simulink model "second_order_DDPG_change_obs"  (R2024a)
settings: Solver=FixedStepAuto  StartTime=0.0  StopTime=500  FixedStep=0.001  RelTol=1e-3
libraries: rllib x1, simulink x1
settings Model: Creator=Steven  LastModifiedBy=Steven
settings DebuggingCC: UnconnectedInputMsg=warning  UnconnectedOutputMsg=warning  UnconnectedLineMsg=warning
settings ModelReferenceCC: EnableRefExpFcnMdlSchedulingChecks=on
settings RTWCC: GPUComputeCapability=3.5  DLArmComputeVersion=19.05

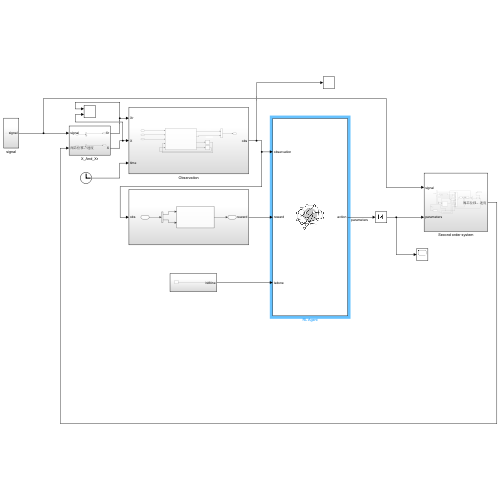
[thumbnail: Simulink's stored preview of the top-level diagram]
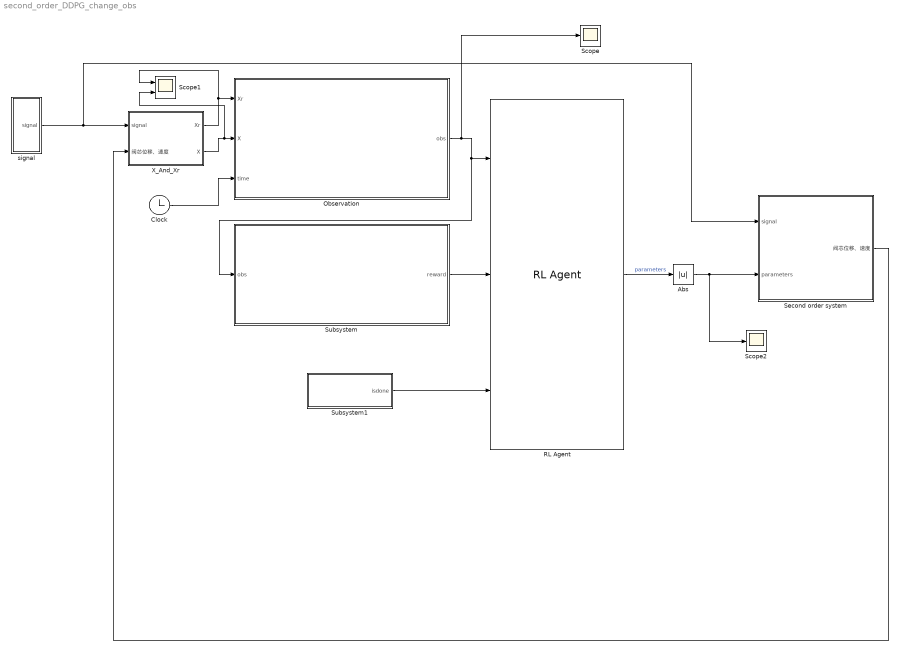
== system second_order_DDPG_change_obs ==
  Abs : Abs  SaturateOnIntegerOverflow=off
  Clock : Clock
  Observation : Subsystem
  RL Agent : rllib/RL Agent  Agent=agent_second_order  ExternalActionAsInput=off  ProvideLastAction=off  ProvideCumRwd=off  TreatAsDirectFeedthrough=on  UseStrictObservationDataTypes=off
  Scope : Scope
  Scope1 : Scope  NumInputPorts=2
  Scope2 : Scope
  Second order system : Subsystem
  Subsystem : Subsystem
  Subsystem1 : Subsystem
  X_And_Xr : Subsystem
  signal : Subsystem
  wires:
  RL Agent/1 -> Abs/1  "parameters"
  signal/1(signal) -> Second order system/1(signal), X_And_Xr/1(signal)
  Second order system/1(阀芯位移、速度) -> X_And_Xr/2(阀芯位移、速度)
  Subsystem1/1(isdone) -> RL Agent/3
  Clock/1 -> Observation/3(time)
  Observation/1(obs) -> Scope/1, Subsystem/1(obs), RL Agent/1
  X_And_Xr/1(Xr) -> Scope1/1, Observation/1(Xr)
  X_And_Xr/2(X) -> Scope1/2, Observation/2(X)
  Subsystem/1(reward) -> RL Agent/2
  Abs/1 -> Scope2/1, Second order system/2(parameters)

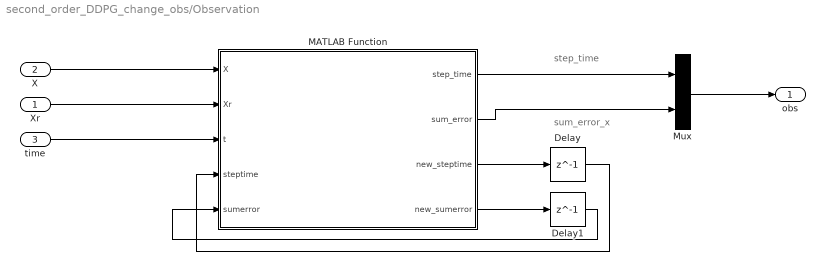
== system second_order_DDPG_change_obs/Observation ==
  note: sum_error_x
  note: step_time
  Xr : Inport
  X : Inport  Port=2
  time : Inport  Port=3
  Delay : Delay  DelayLength=1  InitialCondition=1
  Delay1 : Delay  DelayLength=1  InitialCondition=0
  MATLAB Function : MATLAB Function  TreatAsAtomicUnit=on
  Mux : Mux  Inputs=2
  obs : Outport
  wires:
  MATLAB Function/1(step_time) -> Mux/1
  MATLAB Function/2(sum_error) -> Mux/2
  time/1 -> MATLAB Function/3(t)
  Mux/1 -> obs/1
  Xr/1 -> MATLAB Function/2(Xr)
  X/1 -> MATLAB Function/1(X)
  MATLAB Function/3(new_steptime) -> Delay/1
  Delay/1 -> MATLAB Function/4(steptime)
  MATLAB Function/4(new_sumerror) -> Delay1/1
  Delay1/1 -> MATLAB Function/5(sumerror)

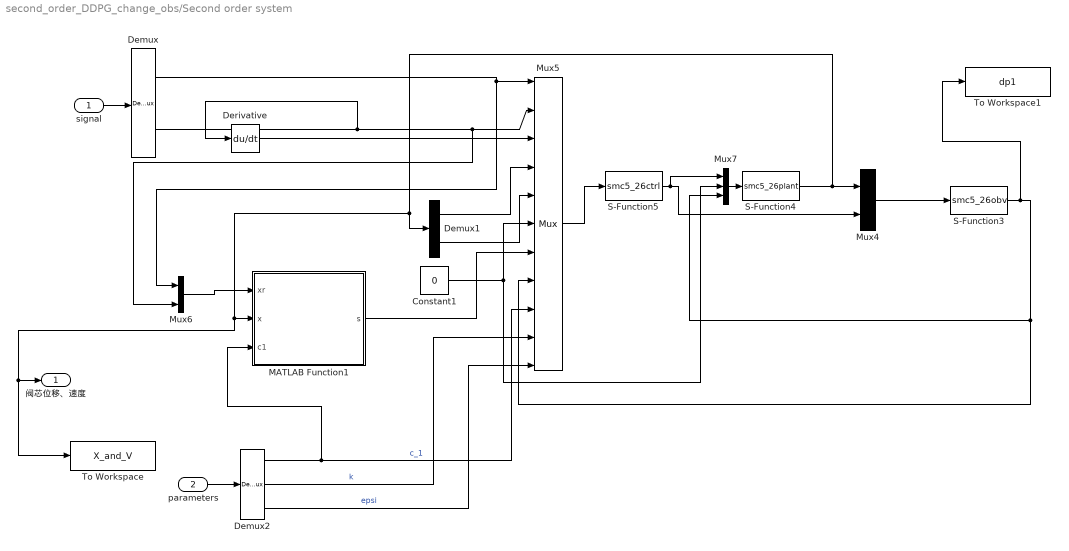
== system second_order_DDPG_change_obs/Second order system ==
  signal : Inport
  parameters : Inport  Port=2
  Constant1 : Constant  Value=0
  Demux : Demux  Outputs=2
  Demux1 : Demux  Outputs=2
  Demux2 : Demux  Outputs=3
  Derivative : Derivative
  MATLAB Function1 : MATLAB Function  TreatAsAtomicUnit=on
  Mux4 : Mux  Inputs=2
  Mux5 : Mux  Inputs=11
  Mux6 : Mux  Inputs=2
  Mux7 : Mux  Inputs=3
  S-Function3 : S-Function  FunctionName=smc5_26obv  SFunctionDeploymentMode=off  EnableBusSupport=off
  S-Function4 : S-Function  FunctionName=smc5_26plant  SFunctionDeploymentMode=off  EnableBusSupport=off
  S-Function5 : S-Function  FunctionName=smc5_26ctrl  SFunctionDeploymentMode=off  EnableBusSupport=off
  To Workspace : ToWorkspace  VariableName=X_and_V  SampleTime=-1
  To Workspace1 : ToWorkspace  VariableName=dp1  SampleTime=-1
      settings: Save2DSignal=2-D array (concatenate along first dimension)
  阀芯位移、速度 : Outport
  wires:
  S-Function3/1 -> To Workspace1/1, Mux7/3, Mux5/8
  Mux5/1 -> S-Function5/1
  Constant1/1 -> Mux7/2, Mux5/6
  MATLAB Function1/1(s) -> Mux5/7
  Demux1/2 -> Mux5/5
  S-Function4/1 -> Demux1/1, To Workspace/1, 阀芯位移、速度/1, MATLAB Function1/2(x), Mux4/1
  Mux4/1 -> S-Function3/1
  Mux6/1 -> MATLAB Function1/1(xr)
  Demux/1 -> Mux6/1, Mux5/1
  Demux1/1 -> Mux5/4
  Mux7/1 -> S-Function4/1
  S-Function5/1 -> Mux7/1, Mux4/2
  signal/1 -> Demux/1
  Demux/2 -> Mux6/2, Mux5/2, Derivative/1
  parameters/1 -> Demux2/1
  Demux2/1 -> MATLAB Function1/3(c1), Mux5/9  "c_1"
  Demux2/2 -> Mux5/10  "k"
  Demux2/3 -> Mux5/11  "epsi"
  Derivative/1 -> Mux5/3

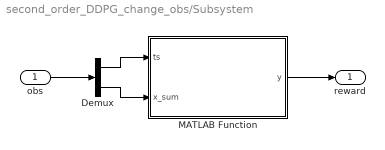
== system second_order_DDPG_change_obs/Subsystem ==
  obs : Inport
  Demux : Demux  Outputs=2
  MATLAB Function : MATLAB Function  TreatAsAtomicUnit=on
  reward : Outport
  wires:
  obs/1 -> Demux/1
  MATLAB Function/1(y) -> reward/1
  Demux/1 -> MATLAB Function/1(ts)
  Demux/2 -> MATLAB Function/2(x_sum)

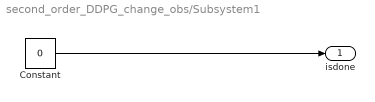
== system second_order_DDPG_change_obs/Subsystem1 ==
  Constant : Constant  Value=0
  isdone : Outport
  wires:
  Constant/1 -> isdone/1

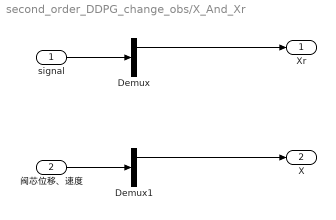
== system second_order_DDPG_change_obs/X_And_Xr ==
  signal : Inport
  阀芯位移、速度 : Inport  Port=2
  Demux : Demux  Outputs=2
  Demux1 : Demux  Outputs=2
  Xr : Outport
  X : Outport  Port=2
  wires:
  signal/1 -> Demux/1
  Demux/1 -> Xr/1
  阀芯位移、速度/1 -> Demux1/1
  Demux1/1 -> X/1

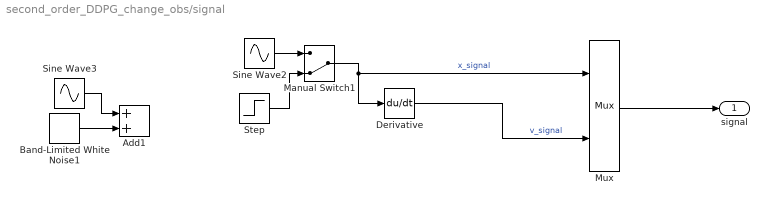
== system second_order_DDPG_change_obs/signal ==
  Add1 : Sum
  Band-Limited White Noise1 : simulink/Sources/Band-Limited White Noise  Cov=[1e-5*1e-5*0.1]  Ts=0.1  seed=[0]
  Derivative : Derivative
  Manual Switch1 : ManualSwitch  CurrentSetting=0
  Mux : Mux  Inputs=2
  Sine Wave2 : Sin  Amplitude=1e-3  Frequency=20*pi  SampleTime=0
  Sine Wave3 : Sin  Amplitude=1e-4  Frequency=30*pi  SampleTime=0
  Step : Step  Time=0  After=1e-4  SampleTime=0
  signal : Outport
  wires:
  Sine Wave2/1 -> Manual Switch1/1
  Step/1 -> Manual Switch1/2
  Manual Switch1/1 -> Mux/1, Derivative/1  "x_signal"
  Derivative/1 -> Mux/2  "v_signal"
  Mux/1 -> signal/1
  Band-Limited White Noise1/1 -> Add1/2
  Sine Wave3/1 -> Add1/1

== matlab function second_order_DDPG_change_obs/Second order system/MATLAB Function1 ==
  data: xr input; s output; x input; c1 input
function s = S(xr,x,c1)
s = c1*(xr(1)-x(1)) + (xr(2)-x(2));

== matlab function second_order_DDPG_change_obs/Observation/MATLAB Function ==
  data: X input; step_time output; Xr input; t input; sum_error output; steptime input; sumerror input; new_steptime output; new_sumerror output
function [step_time, sum_error, new_steptime, new_sumerror] = Calculate_observation(X, Xr, t, steptime, sumerror)
    %计算step_time
    if isempty(steptime)
        steptime = 1;
    end
    Xr_max = 1e-4;
    tolerance = 0.01*Xr_max;
    if abs(X - 0.9*Xr_max) < tolerance
        new_steptime = t;
    else
        new_steptime = steptime;
    end
    step_time = new_steptime;
    
    %计算sum_error
    error = abs(Xr - X);
    if isempty(sumerror)
        sumerror = 0;
    end
    new_sumerror = sumerror + error;
    sum_error = new_sumerror;
end

== matlab function second_order_DDPG_change_obs/Subsystem/MATLAB Function ==
  data: ts input; y output; x_sum input
function y = rewardfunction(ts,x_sum)
c1=50;
c2=200;
y = -(c1*ts+c2*x_sum);
